simulink model "Assembly"  (R2022b)
settings: Solver=FixedStepAuto  StartTime=0.0  StopTime=20  FixedStep=0.001  RelTol=1e-3
model workspace: external: MATLAB File D:\Bw Jiang\Documents\FCS\DuctedFanUAV\Assembly_DataFile.m (data not in the file)
undefined symbols (not defined in the file or in its folder): DiscIntNeverNeededParam, smiData, X, Y, Z
libraries: sm_lib x26, nesl_utility x21, slpidlib x18, simulink_extras x5, simulink x4, shared6dof x2
(part 4 of 4)

== matlab function Assembly/Controller1/Position Controller/Position error transformation (Earth to Body frame) ==
  data: yaw input; xy_err_earth input; xy_err_body output
function xy_err_body = fcn(yaw,xy_err_earth)

transformation = [cos(yaw), sin(yaw); -sin(yaw),  cos(yaw)];
xy_err_body = transformation * xy_err_earth;


end

== matlab function Assembly/Controller/Altitude Controller/D_z1 Function1 ==
  data: err input; u input; y output
function y = fcn(err, u)

% 本函数中的up和down是相对est_Pos中高度值而言的，与实际高度相反
err_abs = abs(err);

gain_far_up = 40;
gain_close_up = 50;
gain_reached_up= 30;

gain_far_down = 60;
gain_close_down = 70;
gain_reached_down= 30;

if err > 0  
    if err_abs > 2
        y = gain_far_up * u;
    elseif err_abs < 1
        y = gain_reached_up * u;
    else
        y = gain_close_up * u;
    end
else
    if err_abs > 2
        y = gain_far_down * u;
    elseif err_abs < 1
        y = gain_reached_down * u;
    else
        y = gain_close_down * u;
    end
end

== matlab function Assembly/角速度转换1 ==
  data: eula input; d_phi output; d_theta output; p input; d_psi output; q input; r input
function [d_phi, d_theta, d_psi] = fcn(eula, p, q, r)

theta = eula(1);
phi = eula(2);
psi = eula(3);

d_phi = p + tan(theta) * sin(phi) * q + tan(theta) * cos(phi) * r;
d_theta = cos(phi) * q - sin(phi) * r;
d_psi = sin(phi) / cos(theta) * q + cos(phi) / cos(theta) * r;

end

== matlab function Assembly/角速度转换2 ==
  data: eula input; p output; q output; d_phi input; r output; d_theta input; d_psi input
function [p, q, r] = fcn(eula, d_phi, d_theta, d_psi)

theta = eula(1);
phi = eula(2);
psi = eula(3);

p = d_phi - sin(theta) * d_psi;
q = cos(phi) * d_theta - cos(theta) * sin(phi) * d_psi;
r = -sin(phi) * d_theta + cos(phi) * cos(theta) * d_psi;

end

== matlab function Assembly/Controller/Position Controller/Error Transform ==
  data: delta_xy_w input; yaw input; delta_xy_b output
function delta_xy_b = fcn(delta_xy_w, yaw)

% 将世界坐标系下x、y方向的偏差变换到机体系下

transformation = [cos(yaw), sin(yaw); -sin(yaw),  cos(yaw)];
delta_xy_b = transformation * delta_xy_w;

end

== matlab function Assembly/力分量/整合力分量 ==
  data: F_total input; fz output; T_yaw input; T_x input; T_y input; tx output; ty output; tz output
function [fz, tx, ty, tz] = fcn(F_total, T_yaw, T_x, T_y)

% 整合为机体坐标系下的F_total、T_yaw、T_x、T_y
% 对于涵道无人机，不需要特殊处理

fz = -F_total;
tx = T_x;
ty = T_y;
tz = T_yaw;

== matlab function Assembly/升力计算器（注意升力计算结果取正值）/升力 ==
  data: n1 input; F_total output; n2 input; T_yaw output
function [F_total, T_yaw] = fcn(n1, n2)

% 总升力取正值
% 假定悬停7000rpm
F_total = (n1 * n1 * 2.414e-7 + n2 * n2 *  2.414e-7) * 2;
T_yaw = (n1 - n2) * 4.65e-8 * 0;

end

== matlab function Assembly/Signal Generator ==
  data: x output; u input; y output; z output; yaw output
function [x, y, z, yaw] = fcn(u)
x = 0;
y = 0;
z = 0;
yaw = 0;
if u <= 0
    x = 0;
    y = 0;
    z = 0;
    yaw = 0;
elseif u - 10 < 0
    x = 0;
    y = 0;
    z = 0;
    yaw = 90*pi/180;
% elseif u - 20 < 0
%     x = 3;
%     y = -1;
%     z = 1;
%     yaw = 0*pi/180;
% elseif u - 30 < 0
%     x = 3;
%     y = -1;
%     z = 0;
%     yaw = 45*pi/180;
end

== matlab function Assembly/World to Body Converter ==
  data: x_0 input; x_b output; y_0 input; z_0 input; y_b output; z_b output; yaw_0 input; yaw_b output
function [x_b, y_b, z_b, yaw_b] = fcn(x_0, y_0, z_0, yaw_0)
x_b = x_0;
y_b = -y_0;
z_b = -z_0;
yaw_b = -yaw_0;
end

== matlab function Assembly/Controller/Yaw Controller/MATLAB Function ==
  data: yaw_ref input; estim_yaw input; err output
function err = fcn(yaw_ref, estim_yaw)

% 全部为弧度制
% 定义三个变量来表达yaw
yaw_ref_n180_p180 = yaw_ref;  % 范围-180~+180
yaw_ref_0_p360 = yaw_ref + pi;  % 范围0~+360
yaw_ref_n360_0 = yaw_ref - pi;  % 范围-360~0

estim_yaw_n180_p180 = estim_yaw;  % 范围-180~+180
estim_yaw_0_p360 = estim_yaw + pi;  % 范围0~+360
estim_yaw_n360_0 = estim_yaw - pi;  % 范围-360~0

if estim_yaw >= 160/180*pi:

== matlab function Assembly/Controller/MATLAB Function ==
  data: x_b0 input; vx_b0 input; x_b output; vx_b output; y_b0 input; vy_b0 input; z_b0 input; vz_b0 input; Q input; y_b output; vy_b output; z_b output; vz_b output
function [x_b, vx_b, y_b, vy_b, z_b, vz_b] = fcn(x_b0, vx_b0, y_b0, vy_b0, z_b0, vz_b0, Q)
